simulink model "RepeatingDownCounter"  (R2023b)
settings: Solver=FixedStepDiscrete  StartTime=0.0  StopTime=0.4  FixedStep=0.01  RelTol=1e-3
settings Model: Creator=Pranav  LastModifiedBy=Pranav

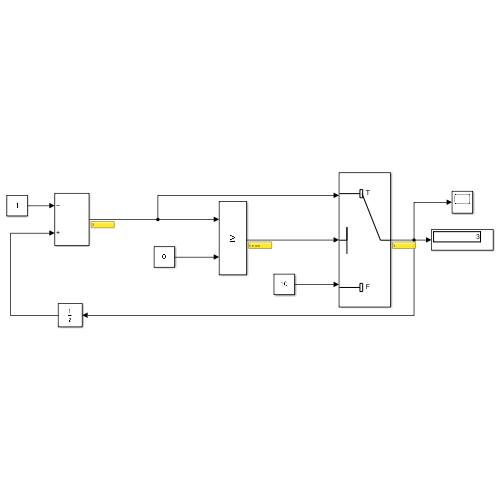
[thumbnail: Simulink's stored preview of the top-level diagram]
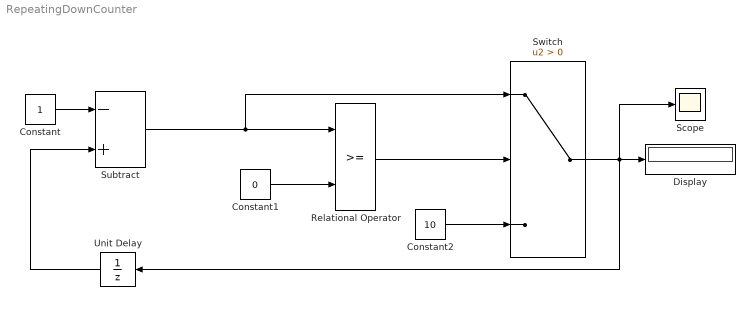
== system RepeatingDownCounter ==
  Constant : Constant
  Constant1 : Constant  Value=0
  Constant2 : Constant  Value=10
  Display : Display
  Relational Operator : RelationalOperator  OutDataTypeStr=boolean  RndMeth=Simplest  InputSameDT=off
  Scope : Scope
  Subtract : Sum  Inputs=-+
  Switch : Switch  Criteria=u2 > Threshold  SaturateOnIntegerOverflow=off  InputSameDT=off
  Unit Delay : UnitDelay  SampleTime=-1  HasFrameUpgradeWarning=on
  wires:
  Relational Operator/1 -> Switch/2
  Switch/1 -> Scope/1, Unit Delay/1, Display/1
  Constant2/1 -> Switch/3
  Constant1/1 -> Relational Operator/2
  Constant/1 -> Subtract/1
  Subtract/1 -> Switch/1, Relational Operator/1
  Unit Delay/1 -> Subtract/2
